simulink model "Einfachsysteme"  (R2021b)
settings: Solver=ode3  StartTime=0.0  StopTime=10.0  FixedStep=0.01  RelTol=1e-3
settings Model: Creator=mwjae  LastModifiedBy=mwjae

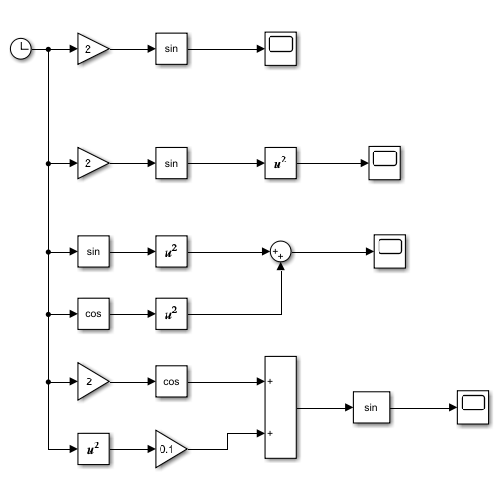
[thumbnail: Simulink's stored preview of the top-level diagram]
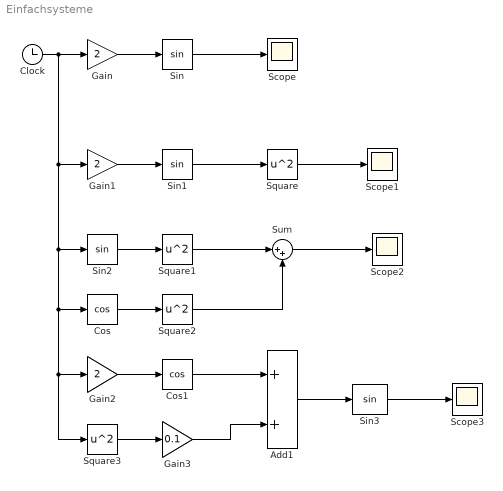
== system Einfachsysteme ==
  Add1 : Sum
  Clock : Clock
  Cos : Trigonometry  Operator=cos
  Cos1 : Trigonometry  Operator=cos
  Gain : Gain  Gain=2
  Gain1 : Gain  Gain=2
  Gain2 : Gain  Gain=2
  Gain3 : Gain  Gain=0.1
  Scope{,1..3} (4 alike) : Scope
  Sin{,1..3} (4 alike) : Trigonometry
  Square{,1..3} (4 alike) : Math  Operator=square  SaturateOnIntegerOverflow=on
  Sum : Sum  Inputs=|++
  wires:
  Gain/1 -> Sin/1
  Sin/1 -> Scope/1
  Clock/1 -> Gain1/1, Square3/1, Gain2/1, Cos/1, Sin2/1, Gain/1
  Gain1/1 -> Sin1/1
  Sin1/1 -> Square/1
  Square/1 -> Scope1/1
  Cos/1 -> Square2/1
  Gain2/1 -> Cos1/1
  Square3/1 -> Gain3/1
  Cos1/1 -> Add1/1
  Gain3/1 -> Add1/2
  Add1/1 -> Sin3/1
  Sin3/1 -> Scope3/1
  Sin2/1 -> Square1/1
  Square1/1 -> Sum/1
  Square2/1 -> Sum/2
  Sum/1 -> Scope2/1
